simulink model "watertank"  (R2018a)
settings: Solver=ode45  StartTime=0.0  StopTime=500.0  RelTol=1e-3  EnableMultiTasking=on
PreLoadFcn:
  | watertankdat
undefined symbols (not defined in the file or in its folder): a, A, b
libraries: fuzblock x1, dspsrcs4 x1
settings Model: Creator=The MathWorks, Inc.  LastModifiedBy=juanje
settings DataIOCC: LimitDataPoints=on  SaveFormat=Array  SignalLoggingName=logsOut
settings OptimizationCC: ExpressionDepthLimit=2147483647  InitFltsAndDblsToZero=on  LifeSpan=inf
settings DebuggingCC: SaveWithParameterizedLinksMsg=none  UnderspecifiedInitializationDetection=Classic  MergeDetectMultiDrivingBlocksExec=none  SignalResolutionControl=TryResolveAllWithWarning  MultiTaskDSMMsg=warning  FcnCallInpInsideContextMsg=warning  AllowSymbolicDim=off  StateNameClashWarn=warning  SFUnexpectedBacktrackingDiag=warning  SFNoUnconditionalDefaultTransitionDiag=warning  SFExecutionAtInitializationDiag=none
settings HardwareCC: ProdBitPerPointer=32  ProdBitPerSizeT=32  ProdBitPerPtrDiffT=32  ProdLargestAtomicFloat=None  ProdIntDivRoundTo=Undefined  ProdEndianess=Unspecified  ProdWordSize=32  ProdHWDeviceType=Specified
settings ModelReferenceCC: PropagateSignalLabelsOutOfModel=off
settings CodeAppCC: StateflowObjectComments=on
settings GRTTargetCC: TargetFcnLib=ansi_tfl_tmw.mat  TargetLangStandard=C89/C90 (ANSI)  GeneratePreprocessorConditionals=Disable all  CombineOutputUpdateFcns=off  GRTInterface=on
settings ConfigComp: CovMetricSettings=dw  CovHtmlReporting=on  CovSaveCumulativeToWorkspaceVar=on  CovSaveSingleToWorkspaceVar=on  CovExternalEMLEnable=off

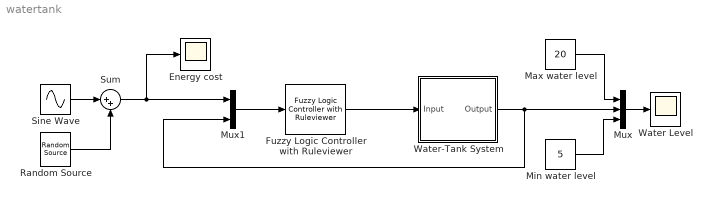
== system watertank ==
  Energy cost : Scope
  Fuzzy Logic Controller with Ruleviewer : fuzblock/Fuzzy Logic  Controller  with Ruleviewer  fismatrix=FIS  Ts=2
  Max water level : Constant  Value=20
  Min water level : Constant  Value=5
  Mux : Mux  Inputs=3
  Mux1 : Mux  Inputs=2
  Random Source : dspsrcs4/Random Source  SrcType=Uniform  NormMethod=Ziggurat  CltLength=12  MinVal=-0.25  MaxVal=0.25  MeanVal=0  VarVal=1  RepMode=Not repeatable  rawSeed=1  IsInherit=off  SampMode=Discrete  SampTime=1  SampFrame=1  DataType=Double  OutComplex=Real  OutputFrames=off
  Sine Wave : Sin  Amplitude=0.5  Bias=1  Frequency=0.1  SampleTime=0
  Sum : Sum  Inputs=|++
  Water Level : Scope
  Water-Tank System : Subsystem
  wires:
  Fuzzy Logic Controller with Ruleviewer/1 -> Water-Tank System/1(Input)
  Mux/1 -> Water Level/1
  Min water level/1 -> Mux/3
  Water-Tank System/1(Output) -> Mux1/2, Mux/2
  Max water level/1 -> Mux/1
  Mux1/1 -> Fuzzy Logic Controller with Ruleviewer/1
  Sine Wave/1 -> Sum/1
  Random Source/1 -> Sum/2
  Sum/1 -> Energy cost/1, Mux1/1

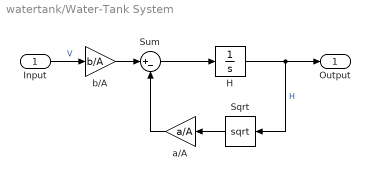
== system watertank/Water-Tank System ==
  Input : Inport
  H : Integrator  InitialCondition=1  LimitOutput=on  LowerSaturationLimit=0
  Sqrt : Sqrt  OutputSignalType=real  SaturateOnIntegerOverflow=on
  Sum : Sum  Inputs=|+-  SaturateOnIntegerOverflow=on
  a/A : Gain  Gain=a/A  SaturateOnIntegerOverflow=on  OutDataTypeStr=Inherit: Same as input  ParamDataTypeStr=Inherit: Same as input
  b/A : Gain  Gain=b/A  SaturateOnIntegerOverflow=on  OutDataTypeStr=Inherit: Same as input  ParamDataTypeStr=Inherit: Same as input
  Output : Outport
  wires:
  b/A/1 -> Sum/1
  Sum/1 -> H/1
  H/1 -> Sqrt/1, Output/1  "H"
  Sqrt/1 -> a/A/1
  a/A/1 -> Sum/2
  Input/1 -> b/A/1  "V"
